simulink model "roll_control_sim_non_linear_velocity"  (R2025b)
settings: Solver=VariableStepAuto  StartTime=0.0  StopTime=15  RelTol=1e-3
values from neighbouring files (symbols this model uses):
  BrasLevier_Set1 = R_tube + Ycp_local_1    (= 0.09)    [setup_main.m]    (also in setup_main_nonLinear.m; setup_main_non_linear_velocity.m)
  BrasLevier_Set2 = R_tube + Ycp_local_2    (= 0.0629791666667)    [setup_main.m]    (also in setup_main_nonLinear.m; setup_main_non_linear_velocity.m)
  BrasLevier_Set3 = R_tube + Ycp_local_3    (= 0.0585717622523)    [setup_main.m]    (also in setup_main_nonLinear.m; setup_main_non_linear_velocity.m)
  Cl_2D_Map = zeros(length(delta_rad_vector), length(Mach_vector))    [setup_main_nonLinear.m]    (also in setup_main_non_linear_velocity.m)
  Cla_Set1 = Cla_iso1 * K_fb1    [setup_main.m]    (also in setup_main_nonLinear.m = Cla_Set1_Static; setup_main_non_linear_velocity.m = Cla_Set1_Static)
  Cla_Set2 = Cla_iso2 * K_fb2    [setup_main.m]    (also in setup_main_nonLinear.m; setup_main_non_linear_velocity.m)
  Cla_Set3 = Cla_iso3 * K_fb3    [setup_main.m]    (also in setup_main_nonLinear.m; setup_main_non_linear_velocity.m)
  Clp_group = Clp_Total_Adim * S_ref * D_tube    [setup_main.m]    (also in setup_main_nonLinear.m = abs(Clp_Total_Adim * S_ref * D_tube); setup_main_non_linear_velocity.m = abs(Clp_Total_Adim * S_ref * D_tube))
  D_tube = 0.10    (= 0.1)    [setup_main.m]    (also in setup_main_nonLinear.m; setup_main_non_linear_velocity.m)
  delta_deg_vector = -30 : 0.5 : 30    [setup_main_nonLinear.m]    (also in setup_main_non_linear_velocity.m)
  I_x = 0.0072    [setup_main.m]    (also in setup_main_nonLinear.m; setup_main_non_linear_velocity.m)
  Kd_data = [0.05, 0.06, 0.06, 0.05, 0.05]    [setup_main.m]    (also in setup_main_nonLinear.m = [8.0, 6.0, 3.0, 1.0, 0.4]; setup_main_non_linear_velocity.m = [0.0, 0.0, 0.0, 0.0, 0.0])
  Ki_data = [2.0, 1.5, 1.0, 0.5, 0.2]    [setup_main.m]    (also in setup_main_nonLinear.m = [0.0, 0.0, 0.0, 0.0, 0.0]; setup_main_non_linear_velocity.m = [5.0, 4.0, 3.0, 1.0, 0.5])
  Kp_data = [6.0, 5.0, 3.5, 2.0, 1.0]    [setup_main.m]    (also in setup_main_nonLinear.m = [12.0, 8.0, 3.0, 1.0, 0.4]; setup_main_non_linear_velocity.m = [8.0, 6.0, 3.0, 1.0, 0.4])
  Mach_vector = 0 : 0.01 : 0.50    [setup_main_nonLinear.m]    (also in setup_main_non_linear_velocity.m)
  q_breakpoints = [ 0, 1000, 3000, 6000, 12000 ]    [setup_main.m]    (also in setup_main_nonLinear.m; setup_main_non_linear_velocity.m)
  rho = 1.18    [setup_main.m]    (also in setup_main_nonLinear.m; setup_main_non_linear_velocity.m)
  S_aileron_Set1 = Set1_Span * (Set1_Cr + Set1_Ct) / 2    (= 0.012)    [setup_main.m]    (also in setup_main_nonLinear.m; setup_main_non_linear_velocity.m)
  S_aileron_Set2 = Set2_Span * (Set2_Cr + Set2_Ct) / 2    (= 0.00896)    [setup_main.m]    (also in setup_main_nonLinear.m; setup_main_non_linear_velocity.m)
  S_aileron_Set3 = Set3_Span * (Set3_Cr + Set3_Ct) / 2    (= 0.000955164)    [setup_main.m]    (also in setup_main_nonLinear.m; setup_main_non_linear_velocity.m)
  S_ref = pi * R_tube^2    (= 0.00785398163397)    [setup_main.m]    (also in setup_main_nonLinear.m; setup_main_non_linear_velocity.m)
  t_motor = [0, 0.1, 0.2, 0.3, 0.4, 0.5, 0.6, 0.7, 0.8, 0.9, 1.0, 1.1, 1.2, 1.3, 1.4, 15.0]    [setup_main_non_linear_velocity.m]
  T_motor = [780.77, 628.21, 583.33, 551.92, 538.46, 529.49, 507.05, 448.72, 403.85, 358.97, 314.10, 197.44, 89.74, 22.44, 0, 0]    [setup_main_non_linear_velocity.m]
  Ts_gyro = 1 / Freq_echantillonnage_Hz    (= 0.01)    [setup_main_non_linear_velocity.m]
undefined symbols (not defined in the file or in its folder): external
libraries: simulink x1, slpidlib x1
settings Model: Creator=theoadam  LastModifiedBy=theoadam

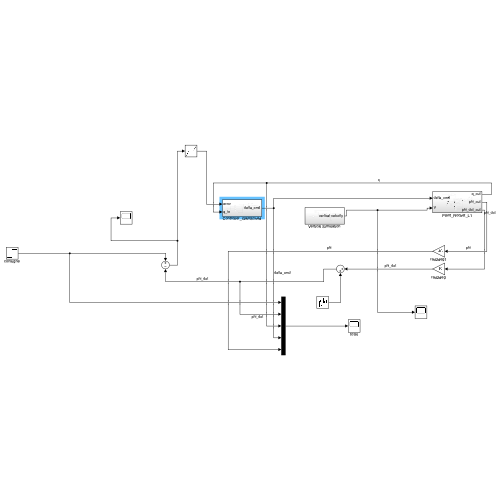
[thumbnail: Simulink's stored preview of the top-level diagram]
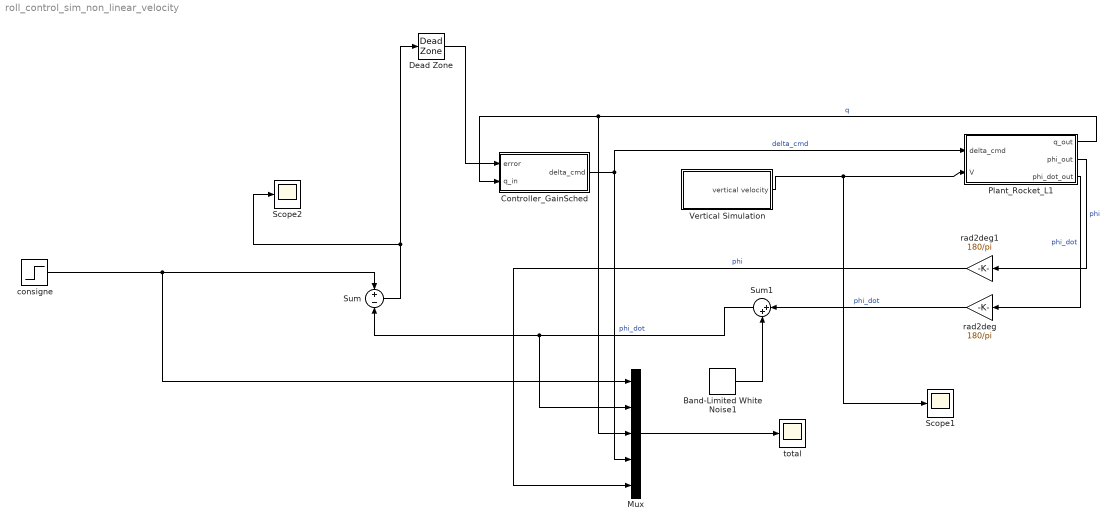
== system roll_control_sim_non_linear_velocity ==
  Band-Limited White Noise1 : simulink/Sources/Band-Limited White Noise  Cov=Gyro_Noise_Power  Ts=Ts_gyro  seed=[23341]
  Controller_GainSched : Subsystem
  Dead Zone : DeadZone  LowerValue=0  UpperValue=0
  Mux : Mux  Inputs=5
  Plant_Rocket_L1 : Subsystem
  Scope1 : Scope
      settings: ActiveDisplayYMinimum=-122.78815768623532  ActiveDisplayYMaximum=161.5459306894661  DataLoggingVariableName=ScopeData6
  Scope2 : Scope
      settings: ActiveDisplayYMinimum=-1  ActiveDisplayYMaximum=1  DataLoggingVariableName=ScopeData7
  Sum : Sum  Inputs=+-
  Sum1 : Sum  Inputs=|++
  Vertical Simulation : Subsystem
  consigne : Step  Time=0  After=0  SampleTime=0
  rad2deg : Gain  Gain=180/pi
  rad2deg1 : Gain  Gain=180/pi
  total : Scope
      settings: ActiveDisplayYMinimum=-29.312733009910318  ActiveDisplayYMaximum=13.912285564434956  DataLoggingVariableName=ScopeData2
  wires:
  consigne/1 -> Mux/1, Sum/1
  Sum/1 -> Dead Zone/1, Scope2/1
  Controller_GainSched/1(delta_cmd) -> Plant_Rocket_L1/1(delta_cmd), Mux/4  "delta_cmd"
  Plant_Rocket_L1/1(q_out) -> Mux/3, Controller_GainSched/2(q_in)  "q"
  Mux/1 -> total/1
  Vertical Simulation/1(vertical velocity) -> Scope1/1, Plant_Rocket_L1/2(V)
  Plant_Rocket_L1/2(phi_out) -> rad2deg1/1  "phi"
  Plant_Rocket_L1/3(phi_dot_out) -> rad2deg/1  "phi_dot"
  Band-Limited White Noise1/1 -> Sum1/2
  Sum1/1 -> Sum/2, Mux/2  "phi_dot"
  rad2deg/1 -> Sum1/1  "phi_dot"
  rad2deg1/1 -> Mux/5  "phi"
  Dead Zone/1 -> Controller_GainSched/1(error)

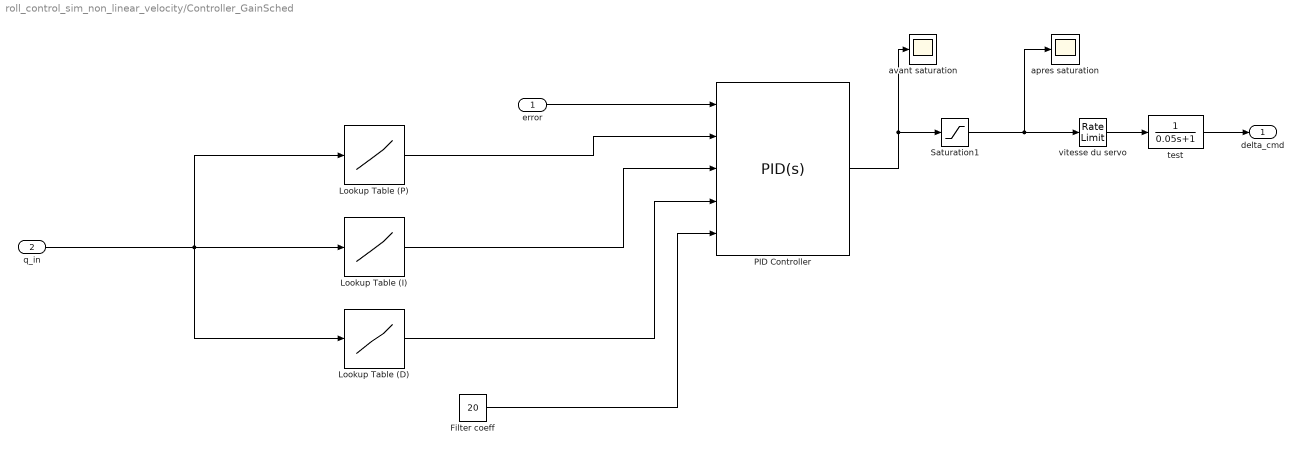
== system roll_control_sim_non_linear_velocity/Controller_GainSched ==
  error : Inport
  q_in : Inport  Port=2
  " test" : TransferFcn  Denominator=[0.05 1]
  Filter coeff : Constant  Value=20
  Lookup Table (D) : Lookup_n-D  NumberOfTableDimensions=1  BreakpointsForDimension1=q_breakpoints  Table=Kd_data  InternalRulePriority=Speed  RndMeth=Simplest
  Lookup Table (I) : Lookup_n-D  NumberOfTableDimensions=1  BreakpointsForDimension1=q_breakpoints  Table=Ki_data  InternalRulePriority=Speed  RndMeth=Simplest
  Lookup Table (P) : Lookup_n-D  NumberOfTableDimensions=1  BreakpointsForDimension1=q_breakpoints  Table=Kp_data  InternalRulePriority=Speed  RndMeth=Simplest
  PID Controller : slpidlib/PID Controller  Controller=PID  Form=Parallel  TimeDomain=Continuous-time  UseExternalTs=off  SampleTime=-1  IntegratorMethod=Forward Euler  FilterMethod=Forward Euler  ControllerParametersSource=external  P=1  I=1  UseKiTs=off  D=0  UseExternalDerivativeSource=off  N=100  UseFilter=on  TunerSelectOption=Transfer Function Based (PID Tuner App)  InitialConditionSource=internal  InitialConditionForIntegrator=0  InitialConditionForFilter=0  DifferentiatorICPrevScaledInput=0  ExternalReset=none  TrackingMode=off  Kt=1  LimitOutput=on  SatLimitsSource=internal  UpperSaturationLimit=15  LowerSaturationLimit=-15  LinearizeAsGain=on  AntiWindupMode=clamping  Kb=external  LimitIntegrator=off  UpperIntegratorSaturationLimit=inf  LowerIntegratorSaturationLimit=-inf  POutMin=[]  POutMax=[]  IOutMin=[]  IOutMax=[]  DOutMin=[]  DOutMax=[]  NOutMin=[]  NOutMax=[]  SumOutMin=[]  SumOutMax=[]  SaturationOutMin=[]  SaturationOutMax=[]  PParamMin=[]  PParamMax=[]  IParamMin=[]  IParamMax=[]  DParamMin=[]  DParamMax=[]  NParamMin=[]  NParamMax=[]  KbParamMin=[]  KbParamMax=[]  KtParamMin=[]  KtParamMax=[]  KbOutMin=[]  KbOutMax=[]  KtOutMin=[]  KtOutMax=[]  IntegratorOutMin=[]  IntegratorOutMax=[]  FilterOutMin=[]  FilterOutMax=[]  SumI1OutMin=[]  SumI1OutMax=[]  SumI2OutMin=[]  SumI2OutMax=[]  SumI3OutMin=[]  SumI3OutMax=[]  SumI4OutMin=[]  SumI4OutMax=[]  SumDOutMin=[]  SumDOutMax=[]  DifferentiatorOutMin=[]  DifferentiatorOutMax=[]  FilterDiffOutCoefMin=[]  FilterDiffOutCoefMax=[]  ReciprocalOutMin=[]  ReciprocalOutMax=[]  SumDenOutMin=[]  SumDenOutMax=[]  SumNumOutMin=[]  SumNumOutMax=[]  DivideOutMin=[]  DivideOutMax=[]  UdiffTsProdOutMin=[]  UdiffTsProdOutMax=[]  NTsProdOutMin=[]  NTsProdOutMax=[]  UintegralTsProdOutMin=[]  UintegralTsProdOutMax=[]  UngainTsProdOutMin=[]  UngainTsProdOutMax=[]  ClampingZeroOutDataTypeStr=Inherit: Inherit via back propagation  ClampingZeroOutMin=[]  ClampingZeroOutMax=[]  FilterDenConstantOutDataTypeStr=Inherit: Inherit via back propagation  FilterDenConstantOutMin=[]  FilterDenConstantOutMax=[]  PCopyOutDataTypeStr=Inherit: Inherit via back propagation  PCopyOutMin=[]  PCopyOutMax=[]  NCopyOutDataTypeStr=Inherit: Inherit via back propagation  NCopyOutMin=[]  NCopyOutMax=[]  IntegratorContinuousStateAttributes=''  IntegratorStateMustResolveToSignalObject=off  IntegratorRTWStateStorageClass=Auto  FilterContinuousStateAttributes=''  FilterStateMustResolveToSignalObject=off  FilterRTWStateStorageClass=Auto  ParallelPVariant=ExternalParameters  IdealPVariant=Disabled  IVariant=ExternalParameters  DVariant=ExternalParameters  IntegratorVariant=Continuous  SatVariant=Enabled  AWVariant=ContClampingParallel  PCopyVariant=Disabled  TRVariant=Disabled  FdbkBlocksVariant=Forward  IdealPFdbkVariant=Disabled  SatFdbkVariant=Disabled  DerivativeFilterVariant=ContFilter  NVariant=ExternalParameters  NCopyVariant=Disabled  FilterICVariant=InternalICsFilter  IntegratorICVariant=InternalICs  ExternalResetVariant=Disabled  TRSumVariant=Passthrough  SumFdbkVariant=Disabled  SumVariant=Sum_PID  TsampFilterVariant=InternalTs  TsampNgainVariant=Passthrough  TsampIntegralVariant=Disabled_SignalSpec  ExternalSaturationOutDataTypeStr=Inherit: Same as second input  DerivativeSourceVariant=ErrorSignal  PreIntVariant=InternalPreInt
  Saturation1 : Saturate  UpperLimit=15  LowerLimit=-15
  apres saturation : Scope
      settings: ActiveDisplayYMinimum=-1  ActiveDisplayYMaximum=1  DataLoggingVariableName=ScopeData8
  avant saturation : Scope
      settings: ActiveDisplayYMinimum=-1744.8133838777017  ActiveDisplayYMaximum=193.868153764189  DataLoggingVariableName=ScopeData5
  vitesse du servo : RateLimiter  RisingSlewLimit=500  FallingSlewLimit=-500  SampleTimeMode=inherited
  delta_cmd : Outport
  wires:
  error/1 -> PID Controller/1
  q_in/1 -> Lookup Table (D)/1, Lookup Table (P)/1, Lookup Table (I)/1
  Lookup Table (P)/1 -> PID Controller/2
  Lookup Table (I)/1 -> PID Controller/3
  Lookup Table (D)/1 -> PID Controller/4
  Filter coeff/1 -> PID Controller/5
  PID Controller/1 -> Saturation1/1, avant saturation/1
  Saturation1/1 -> apres saturation/1, vitesse du servo/1
  vitesse du servo/1 -> " test"/1
  " test"/1 -> delta_cmd/1

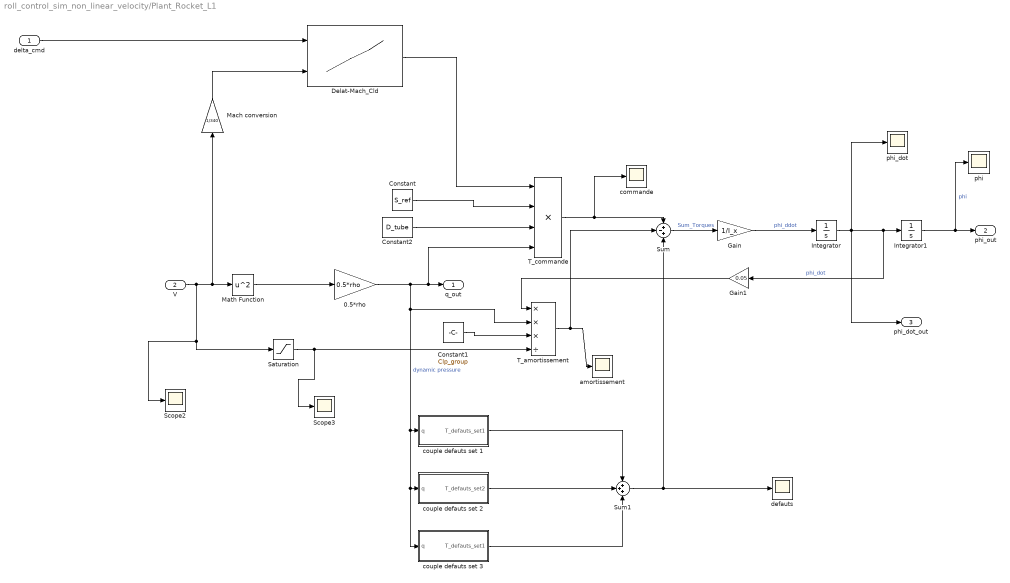
== system roll_control_sim_non_linear_velocity/Plant_Rocket_L1 ==
  delta_cmd : Inport
  V : Inport  Port=2
  0.5*rho : Gain  Gain=0.5*rho
  Constant : Constant  Value=S_ref
  Constant1 : Constant  Value=Clp_group
  Constant2 : Constant  Value=D_tube
  Delat-Mach_Cld : Lookup_n-D  BreakpointsForDimension1=delta_deg_vector  BreakpointsForDimension2=Mach_vector  BreakpointsForDimension3=[5, 7]  Table=Cl_2D_Map  InterpMethod=Cubic spline  ExtrapMethod=Clip  InternalRulePriority=Speed  RndMeth=Simplest
      settings: InputPortMap=u0,u1
  Gain : Gain  Gain=1/I_x
  Gain1 : Gain  Gain=0.05
  Integrator : Integrator
  Integrator1 : Integrator
  Mach conversion : Gain  Gain=1/340
  Math Function : Math  Operator=square
  Saturation : Saturate  UpperLimit=inf  LowerLimit=0.1
  Scope2 : Scope
      settings: ActiveDisplayYMinimum=-1  ActiveDisplayYMaximum=1  DataLoggingVariableName=ScopeData11
  Scope3 : Scope
      settings: ActiveDisplayYMinimum=-0.48102110663534958  ActiveDisplayYMaximum=0.85977375766677611  DataLoggingVariableName=ScopeData12
  Sum : Sum  Inputs=+-+
  Sum1 : Sum  Inputs=+++
  T_amortissement : Product  Inputs=***/
  T_commande : Product  Inputs=4
  amortissement : Scope
      settings: ActiveDisplayYMinimum=-0.017805454900278312  ActiveDisplayYMaximum=0.024523733534271275  DataLoggingVariableName=ScopeData13
  commande : Scope
      settings: ActiveDisplayYMinimum=-0.77633370590278694  ActiveDisplayYMaximum=0.0862593006558652  DataLoggingVariableName=ScopeData4
  couple defauts set 1 : Subsystem
  couple defauts set 2 : Subsystem
  couple defauts set 3 : Subsystem
  defauts : Scope
      settings: ActiveDisplayYMinimum=-0.05861818299451077  ActiveDisplayYMaximum=0.5275636469505971  DataLoggingVariableName=ScopeData14
  phi : Scope
      settings: ActiveDisplayYMinimum=-0.023260564666210157  ActiveDisplayYMaximum=0.20934508199589144  DataLoggingVariableName=ScopeData10
  phi_dot : Scope
      settings: ActiveDisplayYMinimum=-1  ActiveDisplayYMaximum=1  DataLoggingVariableName=ScopeData15
  q_out : Outport
  phi_out : Outport  Port=2
  phi_dot_out : Outport  Port=3
  wires:
  Integrator1/1 -> phi_out/1, phi/1  "phi"
  Integrator/1 -> phi_dot_out/1, phi_dot/1, Gain1/1, Integrator1/1  "phi_dot"
  T_commande/1 -> Sum/1, commande/1
  0.5*rho/1 -> couple defauts set 3/1(q), couple defauts set 2/1(q), couple defauts set 1/1(q), T_amortissement/2, T_commande/4, q_out/1  "dynamic pressure"
  Sum/1 -> Gain/1  "Sum_Torques"
  Gain/1 -> Integrator/1  "phi_ddot"
  Delat-Mach_Cld/1 -> T_commande/1
  Math Function/1 -> 0.5*rho/1
  V/1 -> Scope2/1, Saturation/1, Math Function/1, Mach conversion/1
  Constant1/1 -> T_amortissement/3
  Gain1/1 -> T_amortissement/1
  T_amortissement/1 -> Sum/2, amortissement/1
  Saturation/1 -> Scope3/1, T_amortissement/4
  Sum1/1 -> defauts/1, Sum/3
  couple defauts set 2/1(T_defauts_set2) -> Sum1/2
  couple defauts set 1/1(T_defauts_set1) -> Sum1/1
  couple defauts set 3/1(T_defauts_set1) -> Sum1/3
  delta_cmd/1 -> Delat-Mach_Cld/1
  Constant2/1 -> T_commande/3
  Constant/1 -> T_commande/2
  Mach conversion/1 -> Delat-Mach_Cld/2

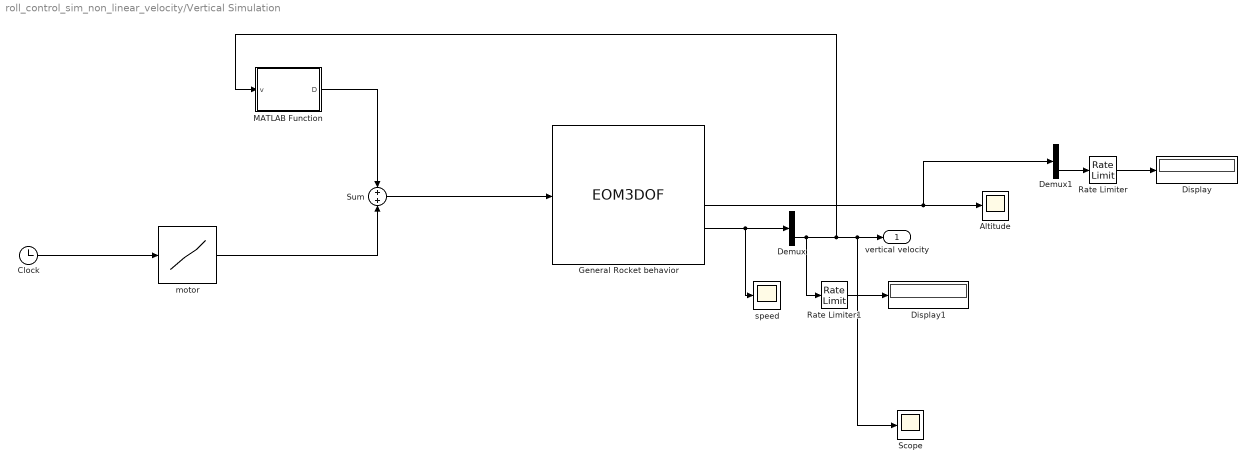
== system roll_control_sim_non_linear_velocity/Vertical Simulation ==
  Altitude : Scope
      settings: ActiveDisplayYMinimum=-93.084002970277311  ActiveDisplayYMaximum=748.76816451948412
  Clock : Clock
  Demux : Demux  Outputs=2
  Demux1 : Demux  Outputs=2
  Display : Display
  Display1 : Display
  General Rocket behavior : EOM3DOF  v_ini=0  mass=3.98  g=-9.81
  MATLAB Function : MATLAB Function  TreatAsAtomicUnit=on
  Rate Limiter : RateLimiter  RisingSlewLimit=99999999  FallingSlewLimit=0  SampleTimeMode=inherited
  Rate Limiter1 : RateLimiter  RisingSlewLimit=99999999  FallingSlewLimit=0  SampleTimeMode=inherited
  Scope : Scope
      settings: ActiveDisplayYMinimum=-1  ActiveDisplayYMaximum=1  DataLoggingVariableName=ScopeData3
  Sum : Sum
  motor : Lookup_n-D  NumberOfTableDimensions=1  BreakpointsForDimension1=t_motor  Table=T_motor  InternalRulePriority=Speed  RndMeth=Simplest
  speed : Scope
      settings: ActiveDisplayYMinimum=-120.04482647954821  ActiveDisplayYMaximum=173.84246704969581
  vertical velocity : Outport
  wires:
  Sum/1 -> General Rocket behavior/2
  General Rocket behavior/5 -> speed/1, Demux/1
  Demux/2 -> Rate Limiter1/1, Scope/1, vertical velocity/1, MATLAB Function/1(v)
  motor/1 -> Sum/2
  General Rocket behavior/4 -> Demux1/1, Altitude/1
  MATLAB Function/1(D) -> Sum/1
  Demux1/2 -> Rate Limiter/1
  Rate Limiter/1 -> Display/1
  Rate Limiter1/1 -> Display1/1
  Clock/1 -> motor/1

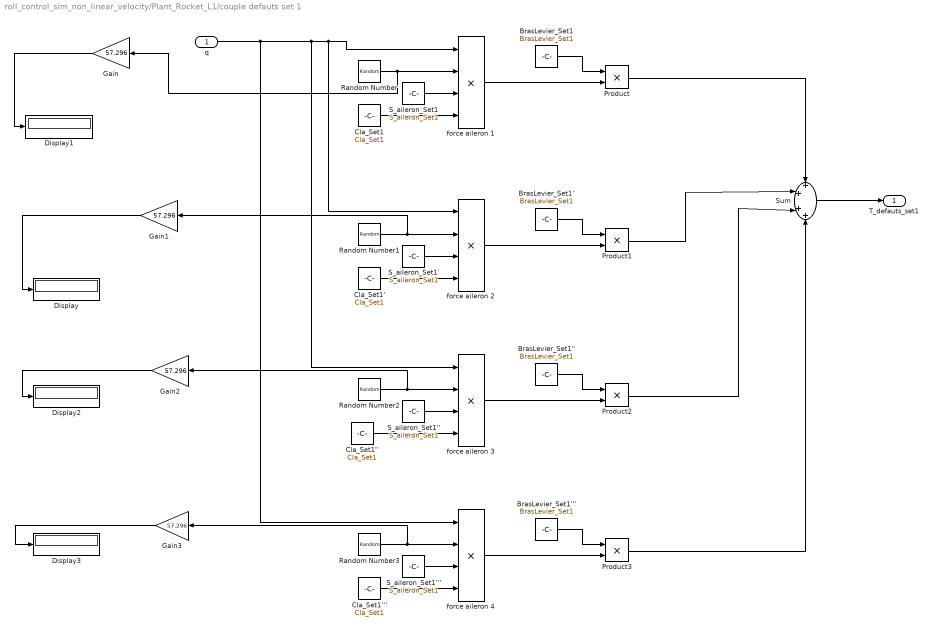
== system roll_control_sim_non_linear_velocity/Plant_Rocket_L1/couple defauts set 1 ==
  q : Inport
  BrasLevier_Set1 : Constant  Value=BrasLevier_Set1
  BrasLevier_Set1' : Constant  Value=BrasLevier_Set1
  BrasLevier_Set1'' : Constant  Value=BrasLevier_Set1
  BrasLevier_Set1''' : Constant  Value=BrasLevier_Set1
  Cla_Set1 : Constant  Value=Cla_Set1
  Cla_Set1' : Constant  Value=Cla_Set1
  Cla_Set1'' : Constant  Value=Cla_Set1
  Cla_Set1''' : Constant  Value=Cla_Set1
  Display{,1..3} (4 alike) : Display
  Gain{,1..3} (4 alike) : Gain  Gain=57.296
  Product{,1..3} (4 alike) : Product
  Random Number : RandomNumber  Variance=0.0003046  Seed=1  SampleTime=1000
  Random Number1 : RandomNumber  Variance=0.0003046  Seed=2  SampleTime=1000
  Random Number2 : RandomNumber  Variance=0.0003046  Seed=3  SampleTime=1000
  Random Number3 : RandomNumber  Variance=0.0003046  Seed=4  SampleTime=1000
  S_aileron_Set1 : Constant  Value=S_aileron_Set1
  S_aileron_Set1' : Constant  Value=S_aileron_Set1
  S_aileron_Set1'' : Constant  Value=S_aileron_Set1
  S_aileron_Set1''' : Constant  Value=S_aileron_Set1
  Sum : Sum  Inputs=++++
  force aileron {1..4} (4 alike) : Product  Inputs=4
  T_defauts_set1 : Outport
  wires:
  Sum/1 -> T_defauts_set1/1
  S_aileron_Set1/1 -> force aileron 1/3
  Cla_Set1/1 -> force aileron 1/4
  force aileron 1/1 -> Product/2
  BrasLevier_Set1/1 -> Product/1
  Product/1 -> Sum/1
  Random Number1/1 -> Gain1/1, force aileron 2/2
  Cla_Set1'/1 -> force aileron 2/4
  Product1/1 -> Sum/2
  force aileron 2/1 -> Product1/2
  BrasLevier_Set1'/1 -> Product1/1
  S_aileron_Set1'/1 -> force aileron 2/3
  Cla_Set1''/1 -> force aileron 3/4
  Product2/1 -> Sum/3
  force aileron 3/1 -> Product2/2
  BrasLevier_Set1''/1 -> Product2/1
  S_aileron_Set1''/1 -> force aileron 3/3
  q/1 -> force aileron 4/1, force aileron 3/1, force aileron 2/1, force aileron 1/1
  Cla_Set1'''/1 -> force aileron 4/4
  Product3/1 -> Sum/4
  force aileron 4/1 -> Product3/2
  BrasLevier_Set1'''/1 -> Product3/1
  S_aileron_Set1'''/1 -> force aileron 4/3
  Random Number/1 -> Gain/1, force aileron 1/2
  Random Number2/1 -> Gain2/1, force aileron 3/2
  Random Number3/1 -> Gain3/1, force aileron 4/2
  Gain/1 -> Display1/1
  Gain1/1 -> Display/1
  Gain2/1 -> Display2/1
  Gain3/1 -> Display3/1

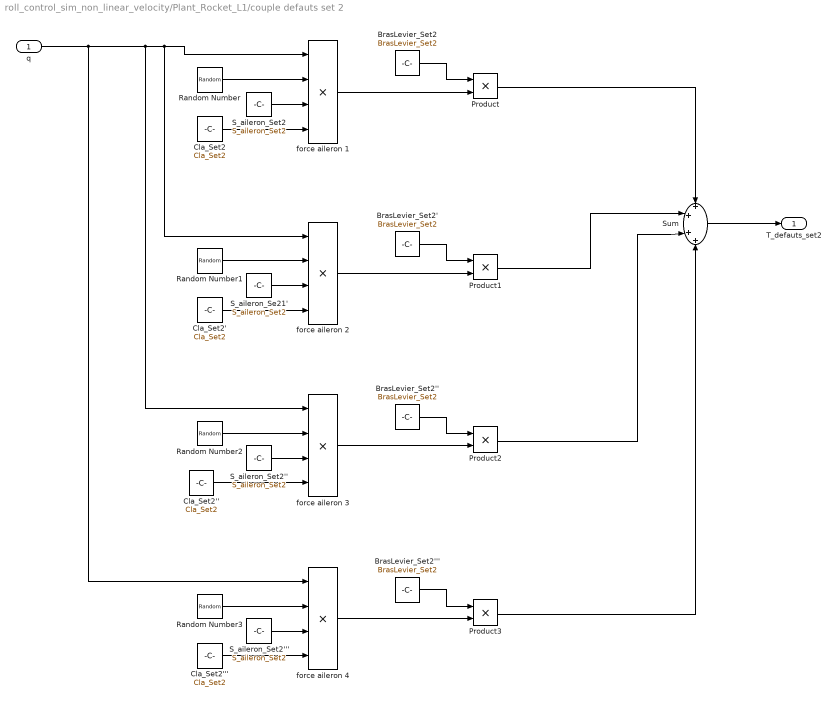
== system roll_control_sim_non_linear_velocity/Plant_Rocket_L1/couple defauts set 2 ==
  q : Inport
  BrasLevier_Set2 : Constant  Value=BrasLevier_Set2
  BrasLevier_Set2' : Constant  Value=BrasLevier_Set2
  BrasLevier_Set2'' : Constant  Value=BrasLevier_Set2
  BrasLevier_Set2''' : Constant  Value=BrasLevier_Set2
  Cla_Set2 : Constant  Value=Cla_Set2
  Cla_Set2' : Constant  Value=Cla_Set2
  Cla_Set2'' : Constant  Value=Cla_Set2
  Cla_Set2''' : Constant  Value=Cla_Set2
  Product{,1..3} (4 alike) : Product
  Random Number : RandomNumber  Variance=0.0003046  Seed=1  SampleTime=1000
  Random Number1 : RandomNumber  Variance=0.0003046  Seed=2  SampleTime=1000
  Random Number2 : RandomNumber  Variance=0.0003046  Seed=3  SampleTime=1000
  Random Number3 : RandomNumber  Variance=0.0003046  Seed=4  SampleTime=1000
  S_aileron_Se21' : Constant  Value=S_aileron_Set2
  S_aileron_Set2 : Constant  Value=S_aileron_Set2
  S_aileron_Set2'' : Constant  Value=S_aileron_Set2
  S_aileron_Set2''' : Constant  Value=S_aileron_Set2
  Sum : Sum  Inputs=++++
  force aileron {1..4} (4 alike) : Product  Inputs=4
  T_defauts_set2 : Outport
  wires:
  Sum/1 -> T_defauts_set2/1
  Random Number/1 -> force aileron 1/2
  S_aileron_Set2/1 -> force aileron 1/3
  Cla_Set2/1 -> force aileron 1/4
  force aileron 1/1 -> Product/2
  BrasLevier_Set2/1 -> Product/1
  Product/1 -> Sum/1
  Random Number1/1 -> force aileron 2/2
  Cla_Set2'/1 -> force aileron 2/4
  Product1/1 -> Sum/2
  force aileron 2/1 -> Product1/2
  BrasLevier_Set2'/1 -> Product1/1
  S_aileron_Se21'/1 -> force aileron 2/3
  Random Number2/1 -> force aileron 3/2
  Cla_Set2''/1 -> force aileron 3/4
  Product2/1 -> Sum/3
  force aileron 3/1 -> Product2/2
  BrasLevier_Set2''/1 -> Product2/1
  S_aileron_Set2''/1 -> force aileron 3/3
  q/1 -> force aileron 4/1, force aileron 3/1, force aileron 2/1, force aileron 1/1
  Random Number3/1 -> force aileron 4/2
  Cla_Set2'''/1 -> force aileron 4/4
  Product3/1 -> Sum/4
  force aileron 4/1 -> Product3/2
  BrasLevier_Set2'''/1 -> Product3/1
  S_aileron_Set2'''/1 -> force aileron 4/3

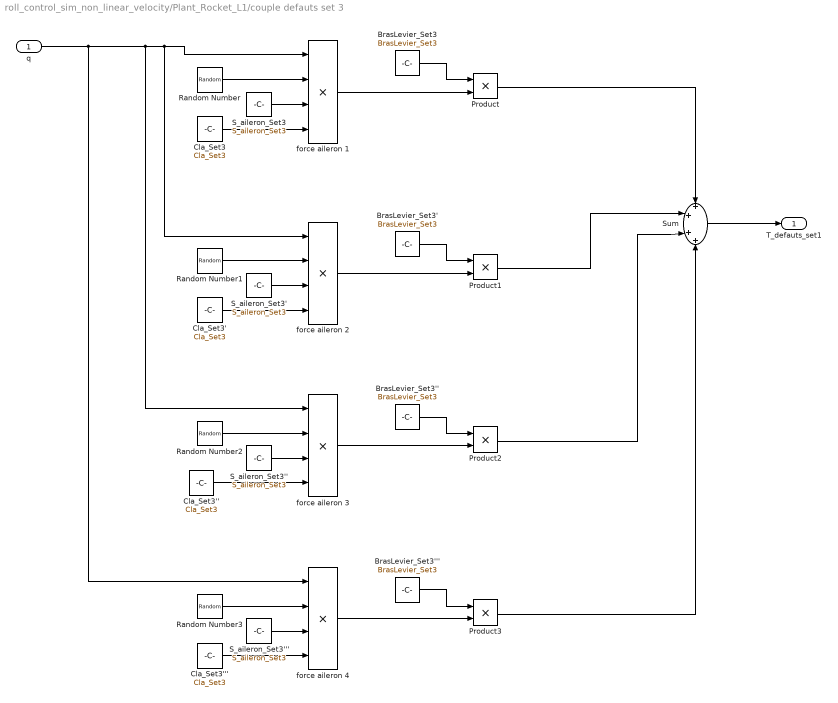
== system roll_control_sim_non_linear_velocity/Plant_Rocket_L1/couple defauts set 3 ==
  q : Inport
  BrasLevier_Set3 : Constant  Value=BrasLevier_Set3
  BrasLevier_Set3' : Constant  Value=BrasLevier_Set3
  BrasLevier_Set3'' : Constant  Value=BrasLevier_Set3
  BrasLevier_Set3''' : Constant  Value=BrasLevier_Set3
  Cla_Set3 : Constant  Value=Cla_Set3
  Cla_Set3' : Constant  Value=Cla_Set3
  Cla_Set3'' : Constant  Value=Cla_Set3
  Cla_Set3''' : Constant  Value=Cla_Set3
  Product{,1..3} (4 alike) : Product
  Random Number : RandomNumber  Variance=0.0003046  Seed=1  SampleTime=1000
  Random Number1 : RandomNumber  Variance=0.0003046  Seed=2  SampleTime=1000
  Random Number2 : RandomNumber  Variance=0.0003046  Seed=3  SampleTime=1000
  Random Number3 : RandomNumber  Variance=0.0003046  Seed=4  SampleTime=1000
  S_aileron_Set3 : Constant  Value=S_aileron_Set3
  S_aileron_Set3' : Constant  Value=S_aileron_Set3
  S_aileron_Set3'' : Constant  Value=S_aileron_Set3
  S_aileron_Set3''' : Constant  Value=S_aileron_Set3
  Sum : Sum  Inputs=++++
  force aileron {1..4} (4 alike) : Product  Inputs=4
  T_defauts_set1 : Outport
  wires:
  Sum/1 -> T_defauts_set1/1
  Random Number/1 -> force aileron 1/2
  S_aileron_Set3/1 -> force aileron 1/3
  Cla_Set3/1 -> force aileron 1/4
  force aileron 1/1 -> Product/2
  BrasLevier_Set3/1 -> Product/1
  Product/1 -> Sum/1
  Random Number1/1 -> force aileron 2/2
  Cla_Set3'/1 -> force aileron 2/4
  Product1/1 -> Sum/2
  force aileron 2/1 -> Product1/2
  BrasLevier_Set3'/1 -> Product1/1
  S_aileron_Set3'/1 -> force aileron 2/3
  Random Number2/1 -> force aileron 3/2
  Cla_Set3''/1 -> force aileron 3/4
  Product2/1 -> Sum/3
  force aileron 3/1 -> Product2/2
  BrasLevier_Set3''/1 -> Product2/1
  S_aileron_Set3''/1 -> force aileron 3/3
  q/1 -> force aileron 4/1, force aileron 3/1, force aileron 2/1, force aileron 1/1
  Random Number3/1 -> force aileron 4/2
  Cla_Set3'''/1 -> force aileron 4/4
  Product3/1 -> Sum/4
  force aileron 4/1 -> Product3/2
  BrasLevier_Set3'''/1 -> Product3/1
  S_aileron_Set3'''/1 -> force aileron 4/3

== matlab function roll_control_sim_non_linear_velocity/Vertical Simulation/MATLAB Function ==
  data: v input; D output
function D = DragForce(v)


A = 0.007854;
C_d = 0.53;
rho = 1.18;



D = -0.5*C_d*rho*A*(v^2); 


end
